simulink model "Ramp"  (R2019b)
settings: Solver=FixedStepAuto  StartTime=0.0  StopTime=6  FixedStep=0.005  RelTol=1e-3
InitFcn:
  | Project_Simulink_Params_April15
values from neighbouring files (symbols this model uses):
  RampEnd = cosd(Angle)* RampLength/V + RampStart    [Project_Simulink_Params_April15.m]
  RampStart = 2    [Project_Simulink_Params_April15.m]
  Slope = tand(1.2*Angle)*V    [Project_Simulink_Params_April15.m]
  V = Vs(i)    [Project_Simulink_Params_April15.m]
libraries: simulink x3
settings Model: Creator=Jordan  LastModifiedBy=Jordan
settings DataIOCC: SaveFormat=Array

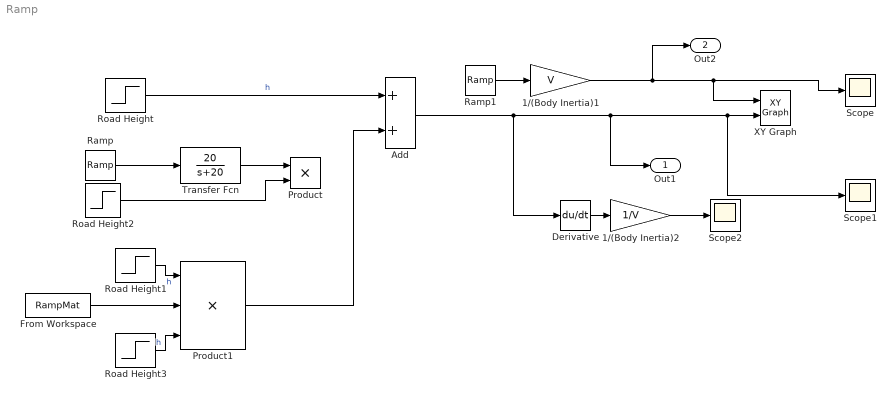
== system Ramp ==
  1/(Body Inertia)1 : Gain  Gain=V  SaturateOnIntegerOverflow=on  OutDataTypeStr=Inherit: Same as input  ParamDataTypeStr=Inherit: Same as input
  1/(Body Inertia)2 : Gain  Gain=1/V  SaturateOnIntegerOverflow=on  OutDataTypeStr=Inherit: Same as input  ParamDataTypeStr=Inherit: Same as input
  Add : Sum
  Derivative : Derivative
  From Workspace : FromWorkspace  VariableName=RampMat  OutputAfterFinalValue=Holding final value
  Product : Product
  Product1 : Product  Inputs=3
  Ramp : simulink/Sources/Ramp  slope=Slope  start=RampStart  InitialOutput=0
  Ramp1 : simulink/Sources/Ramp  slope=1  start=0  InitialOutput=0
  Road Height : Step  Time=0  After=0  SampleTime=0
  Road Height1 : Step  Time=RampStart  SampleTime=0
  Road Height2 : Step  Time=RampEnd  Before=1  After=0  SampleTime=0
  Road Height3 : Step  Time=RampEnd  Before=1  After=0  SampleTime=0
  Scope : Scope
  Scope1 : Scope
  Scope2 : Scope
  Transfer Fcn : TransferFcn  Numerator=[20]  Denominator=[1 20]
  XY Graph : simulink/Sinks/XY Graph  xmin=0  xmax=2  ymin=0  ymax=1  st=-1
  Out1 : Outport
  Out2 : Outport  Port=2
  wires:
  Transfer Fcn/1 -> Product/1
  Road Height/1 -> Add/1  "h"
  Ramp/1 -> Transfer Fcn/1
  Road Height2/1 -> Product/2
  Ramp1/1 -> 1/(Body Inertia)1/1
  1/(Body Inertia)1/1 -> Out2/1, Scope/1, XY Graph/1
  Add/1 -> Derivative/1, Out1/1, Scope1/1, XY Graph/2
  Derivative/1 -> 1/(Body Inertia)2/1
  1/(Body Inertia)2/1 -> Scope2/1
  Road Height1/1 -> Product1/1  "h"
  From Workspace/1 -> Product1/2
  Road Height3/1 -> Product1/3  "h"
  Product1/1 -> Add/2
